simulink model "untitled"  (R2024b)
settings: Solver=VariableStepAuto  StartTime=0.0  StopTime=4  FixedStep=0.05  RelTol=1e-3
values from neighbouring files (symbols this model uses):
  x0 = [ pN1; vN1; pE1; vE1; pD1; vD1; phi1; p1; theta1; q1; psi1; r1;         pN2; vN2; pE2; vE2; pD2; vD2; phi2; p2; theta2; q2; psi2; r2;         start_Np; start_vNp; start_Ep; start_vEp; start_Dp; start_vDp ]    [initial_conditions.m]
settings Model: Creator=alvinisac  LastModifiedBy=alvinisac

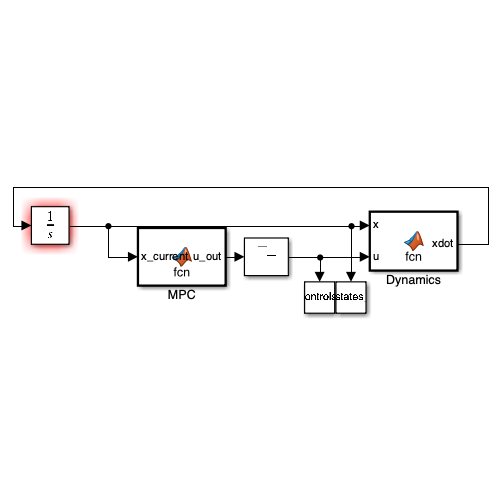
[thumbnail: Simulink's stored preview of the top-level diagram]
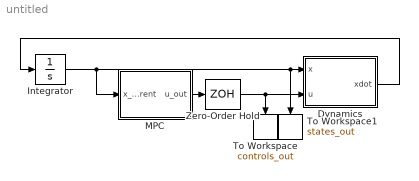
== system untitled ==
  Dynamics : MATLAB Function  TreatAsAtomicUnit=on
  Integrator : Integrator  InitialCondition=x0
  MPC : MATLAB Function  TreatAsAtomicUnit=on  SystemSampleTime=0.05
  To Workspace : ToWorkspace  VariableName=controls_out  SampleTime=0.001
      settings: Save2DSignal=2-D array (concatenate along first dimension)
  To Workspace1 : ToWorkspace  VariableName=states_out  SampleTime=-1
  Zero-Order Hold : ZeroOrderHold  SampleTime=-1
  wires:
  Dynamics/1(xdot) -> Integrator/1
  Integrator/1 -> MPC/1(x_current), Dynamics/1(x), To Workspace1/1
  MPC/1(u_out) -> Zero-Order Hold/1
  Zero-Order Hold/1 -> To Workspace/1, Dynamics/2(u)

== matlab function untitled/MPC ==
  settings: updateMethod=DISCRETE
  data: x_current input; u_out output
function u_out = fcn(x_current)

u_out = mpc_controller_2uav(x_current);

end

== matlab function untitled/Dynamics ==
  settings: updateMethod=DISCRETE
  data: xdot output; x input; u input
function xdot = fcn(x, u)
    xdot = continuous_dynamics_2uav(x, u);
end
